simulink model "SimulinkSampleEncoder"  (R2019a)
settings: Solver=FixedStepDiscrete  StartTime=0.0  StopTime=30  FixedStep=0.01  RelTol=1e-3
undefined symbols (not defined in the file or in its folder): serial
libraries: instrumentlib x2
settings Model: Creator=go_71  LastModifiedBy=Eureka Dynamics
settings DataIOCC: ReturnWorkspaceOutputs=off
settings DebuggingCC: ArithmeticOperatorsInVariantConditions=warning
settings SFSimCC: SimUseLocalCustomCode=off
settings RTWCC: RTWUseLocalCustomCode=off

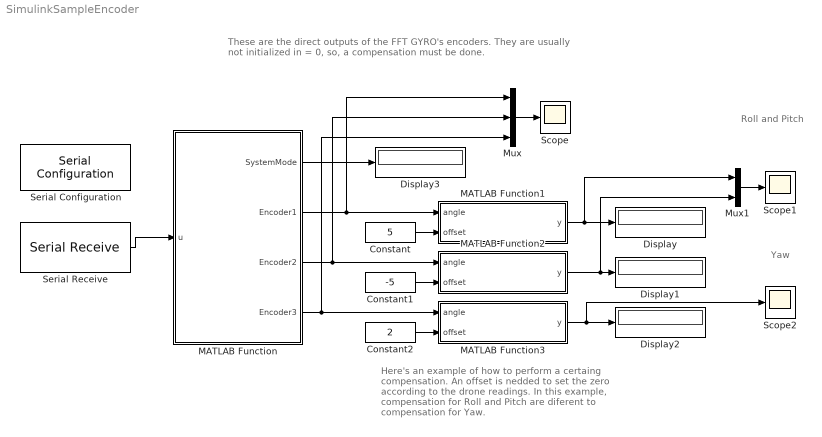
== system SimulinkSampleEncoder ==
  note: Yaw
  note: Roll and Pitch
  note: Here's an example of how to perform a certaing compensation. An offset is nedded to set the zero according to the drone readings.
      | In this example, compensation for Roll and Pitch are diferent to compensation for Yaw.
  note: These are the direct outputs of the FFT GYRO's encoders. They are usually not initialized in = 0, so, a compensation must be done.
  Constant : Constant  Value=5
  Constant1 : Constant  Value=-5
  Constant2 : Constant  Value=2
  Display{,1..3} (4 alike) : Display
  MATLAB Function : MATLAB Function  TreatAsAtomicUnit=on
  MATLAB Function1 : MATLAB Function  TreatAsAtomicUnit=on
  MATLAB Function2 : MATLAB Function  TreatAsAtomicUnit=on
  MATLAB Function3 : MATLAB Function  TreatAsAtomicUnit=on
  Mux : Mux  Inputs=3
  Mux1 : Mux  Inputs=2
  Scope : Scope
  Scope1 : Scope
  Scope2 : Scope
  Serial Configuration : instrumentlib/Serial Configuration  Priority=-200000  ComPortMenu=COM4  ComPort=COM4  ObjConstructor=serial('COM4');  BaudRate=9600  DataBits=8  Parity=none  StopBits=1  FlowControl=none  Timeout=0.05  ByteOrder=LittleEndian
  Serial Receive : instrumentlib/Serial Receive  ComPortMenu=COM4  ComPort=COM4  ObjConstructor=serial('COM4');  Terminator=<none>  DataSize="[32   1]"  DataType=uint8  EnableBlockingMode=on  ActionDataUnavailable=Output last received value  CustomValue=0  SampleTime=0.01
  wires:
  Serial Receive/1 -> MATLAB Function/1(u)
  MATLAB Function/1(SystemMode) -> Display3/1
  Mux/1 -> Scope/1
  MATLAB Function/3(Encoder2) -> MATLAB Function2/1(angle), Mux/2
  MATLAB Function/2(Encoder1) -> MATLAB Function1/1(angle), Mux/1
  MATLAB Function/4(Encoder3) -> MATLAB Function3/1(angle), Mux/3
  MATLAB Function1/1(y) -> Mux1/1, Display/1
  Constant/1 -> MATLAB Function1/2(offset)
  MATLAB Function2/1(y) -> Mux1/2, Display1/1
  Constant1/1 -> MATLAB Function2/2(offset)
  MATLAB Function3/1(y) -> Scope2/1, Display2/1
  Constant2/1 -> MATLAB Function3/2(offset)
  Mux1/1 -> Scope1/1

== matlab function SimulinkSampleEncoder/MATLAB Function1 ==
  data: angle input; y output; offset input
function y = normalizeAngle(angle,offset)

angle = angle - offset;
if angle<0
    y = angle+360;
else
    y = angle;
end

if y>180
    y=y-360;
end
y=-y;

== matlab function SimulinkSampleEncoder/MATLAB Function ==
  data: u input; SystemMode output; Encoder1 output; Encoder2 output; Encoder3 output
function  [SystemMode,Encoder1,Encoder2,Encoder3] = ReadPacketEncoders(u)
%Read Motor Paquet
coder.extrinsic('extractBetween'); 
coder.extrinsic('str2double'); 

SystemMode = 0;
Encoder1=0;
Encoder2=0;
Encoder3=0;

SystemMode = double(uint8(u(2,1)));   %1:Motor   2:Encoder

%PositionM1: byte 5 al 12
PositionE1_aux = char(u(5:12,:));
Encoder1 = str2double(PositionE1_aux');  %str2double( char(u(5:12,:))');
        
%PositionM1: byte 14 al 21
PositionE2_aux = char(u(14:21,:));
Encoder2 = str2double(PositionE2_aux');

%PositionM1: byte 23 al 30
PositionE3_aux = char(u(23:30,:));
Encoder3 = str2double(PositionE3_aux');

nop=1;

== matlab function SimulinkSampleEncoder/MATLAB Function2 ==
  data: angle input; y output; offset input
function y = normalizeAngle(angle,offset)

angle = angle - offset;
if angle<0
    y = angle+360;
else
    y = angle;
end

if y>180
    y=y-360;
end
y=-y;

== matlab function SimulinkSampleEncoder/MATLAB Function3 ==
  data: angle input; y output; offset input
function y = normalizeAngle(angle,offset)

angle = angle - offset;
if angle<0
    y = angle+360;
else
    y = angle;
end


y=360 - y;
